simulink model "vending_machine"  (R2020b)
settings: Solver=FixedStepDiscrete  StartTime=0.0  StopTime=200  FixedStep=0.1  RelTol=1e-3  EnableMultiTasking=on
settings Model: Creator=abhin  LastModifiedBy=abhin
settings DataIOCC: LimitDataPoints=on  SaveFormat=Array  ReturnWorkspaceOutputs=off

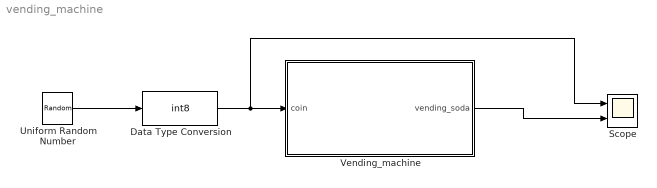
== system vending_machine ==
  Data Type Conversion : DataTypeConversion  OutDataTypeStr=int8  RndMeth=Nearest  SaturateOnIntegerOverflow=on
  Scope : Scope  NumInputPorts=2
  Uniform Random Number : UniformRandomNumber  Maximum=2  Seed=337  SampleTime=10
  Vending_machine : Stateflow chart  TreatAsAtomicUnit=on
  wires:
  Uniform Random Number/1 -> Data Type Conversion/1
  Data Type Conversion/1 -> Scope/1, Vending_machine/1(coin)
  Vending_machine/1(vending_soda) -> Scope/2

== stateflow chart vending_machine/Vending_machine ==
  settings: stateMachineType=MEALY_MACHINE  initializeOutput=1
  state Zero_coin
  state Nickel
  state Dime
  (default) -> Zero_coin
  Zero_coin -> Nickel [order 1] : [coin==1]{vending_soda==0}
  Nickel -> Zero_coin [order 2] : [coin==2]{vending_soda==1}
  Dime -> Zero_coin [order 1] : [coin==1]{vending_soda==0}
  Zero_coin -> Dime [order 2] : [coin==2]{vending_soda==1}
  Nickel -> Dime [order 1] : [coin==1]{vending_soda==0}
  Dime -> Nickel [order 2] : [coin==2]{vending_soda==1}
  data: coin input; vending_soda output
